simulink model "dataGenerator"  (R2019b)
settings: Solver=VariableStepAuto  StartTime=0.0  StopTime=600  RelTol=1e-3
settings Model: Creator=magnus  LastModifiedBy=Afonso

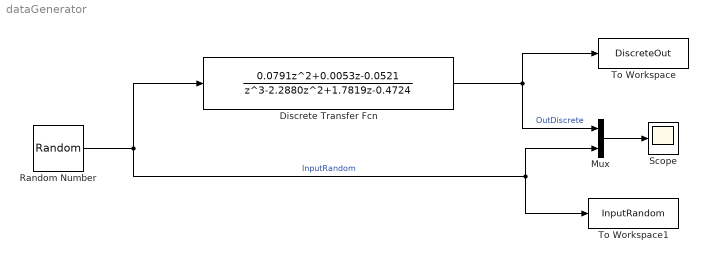
== system dataGenerator ==
  Discrete Transfer Fcn : DiscreteTransferFcn  Numerator=[0 0.0791 0.0053 -0.0521]  Denominator=[1.0000 -2.2880 1.7819 -0.4724]
  Mux : Mux  Inputs=2
  Random Number : RandomNumber  SampleTime=1
  Scope : Scope
  To Workspace : ToWorkspace  VariableName=DiscreteOut  SaveFormat=Timeseries  SampleTime=-1
  To Workspace1 : ToWorkspace  VariableName=InputRandom  SaveFormat=Timeseries  SampleTime=-1
  wires:
  Discrete Transfer Fcn/1 -> To Workspace/1, Mux/1  "OutDiscrete"
  Mux/1 -> Scope/1
  Random Number/1 -> Discrete Transfer Fcn/1, To Workspace1/1, Mux/2  "InputRandom"
